simulink model "MagicFormula"  (R2024b)
settings: Solver=VariableStepAuto  StartTime=0.0  StopTime=10.0  RelTol=1e-3
values from neighbouring files (symbols this model uses):
  B = 10    [magicformulavariables.m]
  C = data{16,2}    [Max_Off_Axis_Rack_F.m]    (also in magicformulavariables.m = 10)
  D = 10    [magicformulavariables.m]
undefined symbols (not defined in the file or in its folder): Bx, Cx, Dx, Ex, Fz
settings Model: Creator=rober  LastModifiedBy=rober

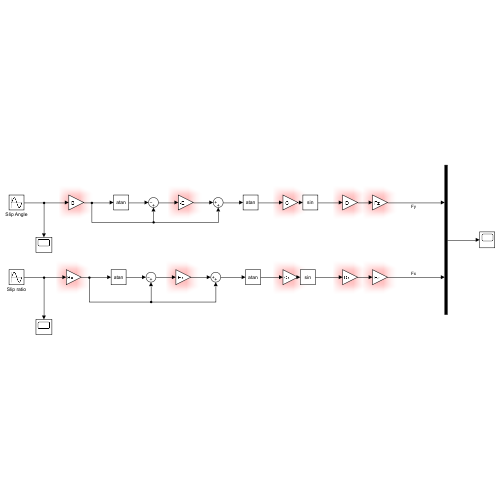
[thumbnail: Simulink's stored preview of the top-level diagram]
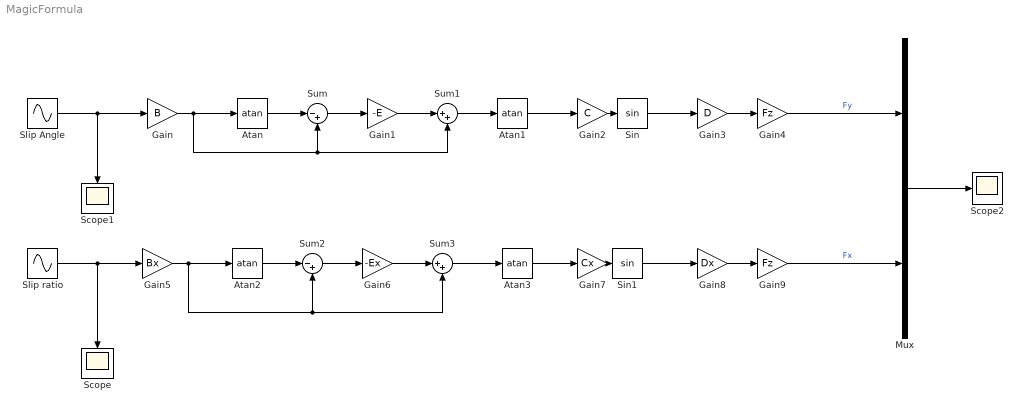
== system MagicFormula ==
  Atan{,1..3} (4 alike) : Trigonometry  Operator=atan
  Gain : Gain  Gain=B
  Gain1 : Gain  Gain=-E
  Gain2 : Gain  Gain=C
  Gain3 : Gain  Gain=D
  Gain4 : Gain  Gain=Fz
  Gain5 : Gain  Gain=Bx
  Gain6 : Gain  Gain=-Ex
  Gain7 : Gain  Gain=Cx
  Gain8 : Gain  Gain=Dx
  Gain9 : Gain  Gain=Fz
  Mux : Mux  Inputs=2
  Scope : Scope
  Scope1 : Scope
  Scope2 : Scope
  Sin : Trigonometry
  Sin1 : Trigonometry
  Slip Angle : Sin  SampleTime=0
  Slip ratio : Sin  SampleTime=0
  Sum : Sum  Inputs=|-+
  Sum1 : Sum  Inputs=|++
  Sum2 : Sum  Inputs=|-+
  Sum3 : Sum  Inputs=|++
  wires:
  Slip Angle/1 -> Gain/1, Scope1/1
  Gain/1 -> Sum1/2, Sum/2, Atan/1
  Atan/1 -> Sum/1
  Sum/1 -> Gain1/1
  Gain1/1 -> Sum1/1
  Sum1/1 -> Atan1/1
  Atan1/1 -> Gain2/1
  Gain2/1 -> Sin/1
  Sin/1 -> Gain3/1
  Gain3/1 -> Gain4/1
  Gain4/1 -> Mux/1  "Fy"
  Atan3/1 -> Gain7/1
  Gain9/1 -> Mux/2  "Fx"
  Gain8/1 -> Gain9/1
  Sin1/1 -> Gain8/1
  Gain5/1 -> Sum3/2, Sum2/2, Atan2/1
  Slip ratio/1 -> Gain5/1, Scope/1
  Atan2/1 -> Sum2/1
  Gain7/1 -> Sin1/1
  Sum3/1 -> Atan3/1
  Sum2/1 -> Gain6/1
  Gain6/1 -> Sum3/1
  Mux/1 -> Scope2/1
